simulink model "chap12_2sim"  (Simulink 8.3)
settings: Solver=ode45  StartTime=0.0  StopTime=40  FixedStep=0.001  RelTol=1e-3
settings Model: Creator=liujk  LastModifiedBy=Administrator  ExtModeTrigMode=oneshot  ExtModeArmWhenConnect=off
settings DataIOCC: LimitDataPoints=off  SignalLoggingName=sigsOut
settings OptimizationCC: BooleanDataType=off
settings DebuggingCC: SaveWithParameterizedLinksMsg=none  SignalResolutionControl=TryResolveAllWithWarning  SolverPrmCheckMsg=none  MultiTaskDSMMsg=warning  MultiTaskCondExecSysMsg=none
settings HardwareCC: TargetUnknown=on
settings RTWCC: IncludeERTFirstTime=on

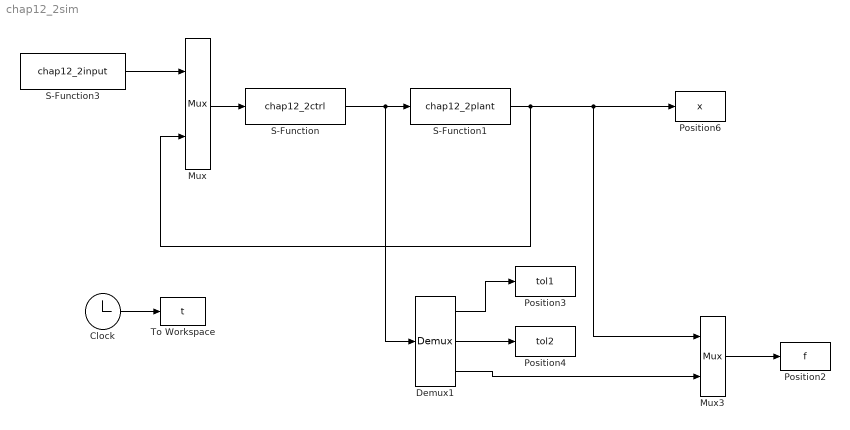
== system chap12_2sim ==
  Clock : Clock
  Demux1 : Demux  Outputs=3
  Mux : Mux  Inputs=2
  Mux3 : Mux  Inputs=2
  Position2 : ToWorkspace  VariableName=f  SampleTime=-1
  Position3 : ToWorkspace  VariableName=tol1  SampleTime=-1
  Position4 : ToWorkspace  VariableName=tol2  SampleTime=-1
  Position6 : ToWorkspace  VariableName=x  SampleTime=-1
  S-Function : S-Function  FunctionName=chap12_2ctrl  EnableBusSupport=off
  S-Function1 : S-Function  FunctionName=chap12_2plant  EnableBusSupport=off
  S-Function3 : S-Function  FunctionName=chap12_2input  EnableBusSupport=off
  To Workspace : ToWorkspace  VariableName=t  SampleTime=-1
  wires:
  Mux/1 -> S-Function/1
  Demux1/1 -> Position3/1
  Demux1/2 -> Position4/1
  S-Function/1 -> S-Function1/1, Demux1/1
  Mux3/1 -> Position2/1
  Demux1/3 -> Mux3/2
  S-Function1/1 -> Mux3/1, Position6/1, Mux/2
  Clock/1 -> To Workspace/1
  S-Function3/1 -> Mux/1
